simulink model "Problem6_DirectForm"  (R2020b)
settings: Solver=VariableStepAuto  StartTime=0.0  StopTime=5  MaxStep=0.01  RelTol=1e-3
settings Model: Creator=vigne  LastModifiedBy=prabhudevmaddipudi

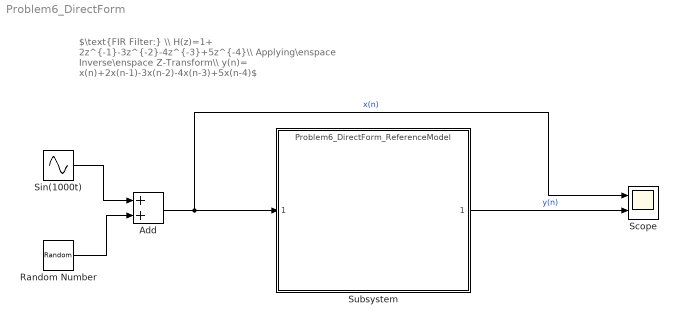
== system Problem6_DirectForm ==
  note: $\text{FIR Filter:} \\ H(z)=1+ 2z^{-1}-3z^{-2}-4z^{-3}+5z^{-4}\\ Applying\enspace Inverse\enspace Z-Transform\\ y(n)= x(n)+2x(n-1)-3x(n-2)-4x(n-3)+5x(n-4)$
  Add : Sum
  Random Number : RandomNumber  SampleTime=0.1
  Scope : Scope  NumInputPorts=2
  Sin(1000t) : Sin  Frequency=2*pi*1000  SampleTime=0
  Subsystem : ModelReference  ModelNameDialog=Problem6_DirectForm_ReferenceModel  SimulationMode=Normal  ModelReferenceVersion=1.2
  wires:
  Sin(1000t)/1 -> Add/1
  Random Number/1 -> Add/2
  Add/1 -> Scope/1, Subsystem/1  "x(n)"
  Subsystem/1 -> Scope/2  "y(n)"
